simulink model "Luo_Converter_with_MOSFET"  (R2025a)
settings: Solver=VariableStepAuto  StartTime=0.0  StopTime=0.5  RelTol=1e-3
libraries: spsMeanLib x16, spsRMSLib x16, spsVoltageMeasurementLib x8, spsCurrentMeasurementLib x7, spsSeriesRLCBranchLib x5, spsDCVoltageSourceLib x1, spsDiodeLib x1, spsMosfetLib x1, sps_lib x1
settings Model: Creator=sanat  LastModifiedBy=sanat

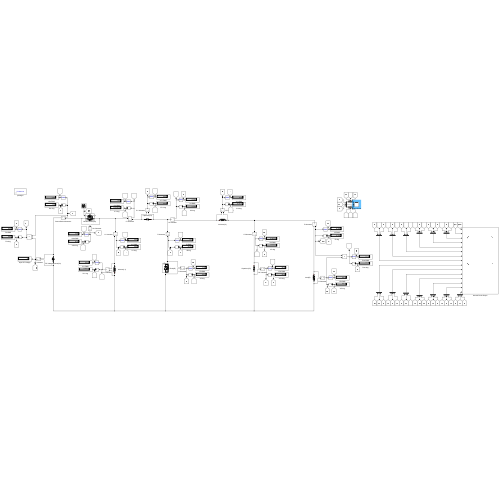
[thumbnail: Simulink's stored preview of the top-level diagram]
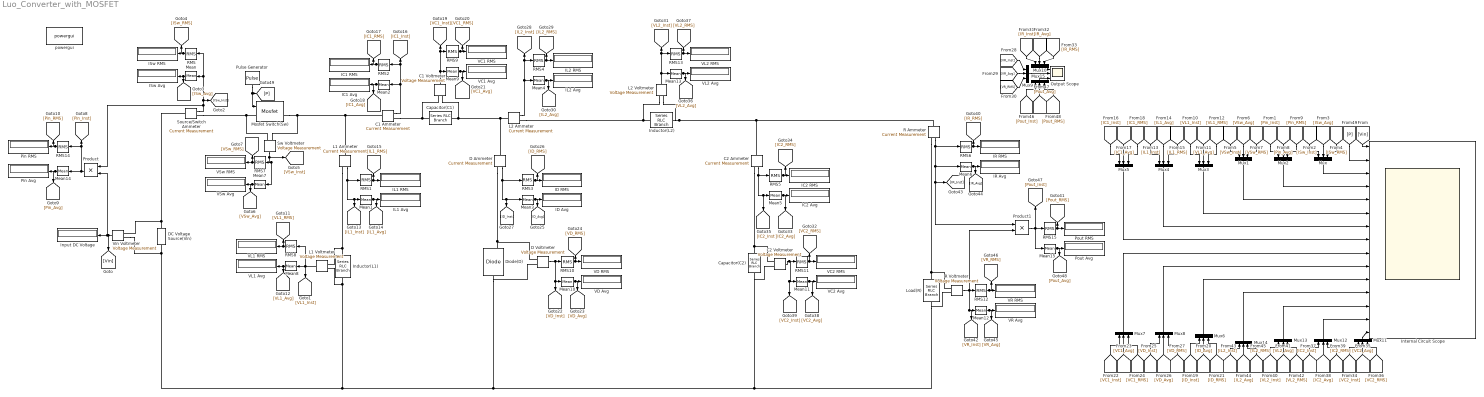
== system Luo_Converter_with_MOSFET ==
  C1 Ammeter : spsCurrentMeasurementLib/Current Measurement  PhasorSimulation=off  OutputType=Complex  PSBequivalent=0
  C1 Voltmeter : spsVoltageMeasurementLib/Voltage Measurement  PhasorSimulation=off  OutputType=Complex  PSBequivalent=0
  C2 Ammeter : spsCurrentMeasurementLib/Current Measurement  PhasorSimulation=off  OutputType=Complex  PSBequivalent=0
  C2 Voltmeter : spsVoltageMeasurementLib/Voltage Measurement  PhasorSimulation=off  OutputType=Complex  PSBequivalent=0
  Capacitor(C1) : spsSeriesRLCBranchLib/Series RLC Branch  LConnTagsString=__new0  RConnTagsString=__new0  BranchType=C  Resistance=1  Inductance=1e-3  SetiL0=off  InitialCurrent=0  Capacitance=21.40e-6  Setx0=off  InitialVoltage=0  Measurements=None
  Capacitor(C2) : spsSeriesRLCBranchLib/Series RLC Branch  LConnTagsString=__new0  RConnTagsString=__new0  BranchType=C  Resistance=1  Inductance=1e-3  SetiL0=off  InitialCurrent=0  Capacitance=30.4e-6  Setx0=off  InitialVoltage=0  Measurements=None
  D Ammeter : spsCurrentMeasurementLib/Current Measurement  PhasorSimulation=off  OutputType=Complex  PSBequivalent=0
  D Voltmeter : spsVoltageMeasurementLib/Voltage Measurement  PhasorSimulation=off  OutputType=Complex  PSBequivalent=0
  DC Voltage Source(Vin) : spsDCVoltageSourceLib/DC Voltage Source  Amplitude=40  Measurements=None
  Diode(D) : spsDiodeLib/Diode  Ron=0.001  Lon=0  Vf=0.8  IC=0  UseSnubber=0  Rs=500  Cs=250e-9  Measurements=on
  IC1 Avg : Display
  IC1 RMS : Display
  IC2 Avg : Display
  IC2 RMS : Display
  ID Avg : Display
  ID RMS : Display
  IL1 Avg : Display
  IL1 RMS : Display
  IL2 Avg : Display
  IL2 RMS : Display
  IR Avg : Display
  IR RMS : Display
  ISw Avg : Display
  ISw RMS : Display
  Inductor(L1) : spsSeriesRLCBranchLib/Series RLC Branch  LConnTagsString=__new0  RConnTagsString=__new0  BranchType=L  Resistance=1  Inductance=36.04e-3  SetiL0=off  InitialCurrent=0  Capacitance=1e-6  Setx0=off  InitialVoltage=0  Measurements=None
  Inductor(L2) : spsSeriesRLCBranchLib/Series RLC Branch  LConnTagsString=__new0  RConnTagsString=__new0  BranchType=L  Resistance=1  Inductance=36.04e-3  SetiL0=off  InitialCurrent=0  Capacitance=1e-6  Setx0=off  InitialVoltage=0  Measurements=None
  Input DC Voltage : Display
  Internal Circuit Scope : Scope  NumInputPorts=15
      settings: ActiveDisplayYMinimum=30  ActiveDisplayYMaximum=50  YLabel=Input Voltage
  L1 Ammeter : spsCurrentMeasurementLib/Current Measurement  PhasorSimulation=off  OutputType=Complex  PSBequivalent=0
  L1 Voltmeter : spsVoltageMeasurementLib/Voltage Measurement  PhasorSimulation=off  OutputType=Complex  PSBequivalent=0
  L2 Ammeter : spsCurrentMeasurementLib/Current Measurement  PhasorSimulation=off  OutputType=Complex  PSBequivalent=0
  L2 Voltmeter : spsVoltageMeasurementLib/Voltage Measurement  PhasorSimulation=off  OutputType=Complex  PSBequivalent=0
  Load(R) : spsSeriesRLCBranchLib/Series RLC Branch  LConnTagsString=__new0  RConnTagsString=__new0  BranchType=R  Resistance=135.2  Inductance=1e-3  SetiL0=off  InitialCurrent=0  Capacitance=1e-6  Setx0=off  InitialVoltage=0  Measurements=None
  Mean{,1..15} (16 alike) : spsMeanLib/Mean  Freq=60  Vinit=0  Ts=0
  Mosfet Switch(Sw) : spsMosfetLib/Mosfet  Ron=0.1  Lon=0  Rd=0.01  Vfd=0  IC=0  Rs=1e5  Cs=inf  Measurements=on
  Mux{,1..15} (16 alike) : Mux  Inputs=3
  Output Scope : Scope  NumInputPorts=3
      settings: ActiveDisplayYMinimum=0.728472  ActiveDisplayYMaximum=0.7284818  YLabel=Resistance(R) Current
  Pin Avg : Display
  Pin RMS : Display
  Pout Avg : Display
  Pout RMS : Display
  Product : Product
  Product1 : Product
  Pulse Generator : DiscretePulseGenerator  PulseType=Time based  Period=1/50000  PulseWidth=(5/7)*100
  R Ammeter : spsCurrentMeasurementLib/Current Measurement  PhasorSimulation=off  OutputType=Complex  PSBequivalent=0
  R Voltmeter : spsVoltageMeasurementLib/Voltage Measurement  PhasorSimulation=off  OutputType=Complex  PSBequivalent=0
  RMS{,1..15} (16 alike) : spsRMSLib/RMS  TrueRMS=on  Freq=60  RMSInit=120  Ts=0
  Source/Switch Ammeter : spsCurrentMeasurementLib/Current Measurement  PhasorSimulation=off  OutputType=Complex  PSBequivalent=0
  Sw Voltmeter : spsVoltageMeasurementLib/Voltage Measurement  PhasorSimulation=off  OutputType=Complex  PSBequivalent=0
  VC1 Avg : Display
  VC1 RMS : Display
  VC2 Avg : Display
  VC2 RMS : Display
  VD Avg : Display
  VD RMS : Display
  VL1 Avg : Display
  VL1 RMS : Display
  VL2 Avg : Display
  VL2 RMS : Display
  VR Avg : Display
  VR RMS : Display
  VSw Avg : Display
  VSw RMS : Display
  Vin Voltmeter : spsVoltageMeasurementLib/Voltage Measurement  PhasorSimulation=off  OutputType=Complex  PSBequivalent=0
  powergui : sps_lib/powergui  Priority=1  SimulationMode=Continuous  SampleTime=50e-6  frequency=60  Iterations=50  frequencyindice=0  Pbase=100e6  ErrMax=1e-4  UnitsV=kV  UnitsW=MW  buscounter=0  FunctionMessages=off  echomessages=off  EnableUseOfTLC=off  CurrentSourceSwitches=off  DisableSnubberDevices=off  DisableRonSwitches=off  DisableVfSwitches=off  DisplayEquations=off  AutomaticDiscreteSolvers=off  SolverType=Tustin/Backward Euler (TBE)  Interpol=off  ExternalGateDelay=off  methode=off  Ts=100  x0status=blocks  SPID=on  SwTol=0  HookPort=off  NonlinearTolerance=1e-4  nMaxIteration=100  ContinueOnMaxIteration=off  RestoreLinks=warning  ResistiveCurrentMeasurement=off  Frange=[0:2:500]  Ylog=off  Xlog=on  ShowGrid=off  save=off  variable=ZData  structure=0  ZoomFFT=off  StartTime=0.0  cycles=1  DisplayStyle=1  fundamental=60  FreqAxis=off  MaxFrequency=1000  frequencyindicesteady=1  RmsSteady=1  display=off
  wires:
  Pulse Generator/1 -> [P], Mosfet Switch(Sw)/1
  Vin Voltmeter/1 -> Product/2, Input DC Voltage/1, [Vin]
  L1 Ammeter/1 -> RMS1/1, [IL1_Inst], Mean1/1
  RMS1/1 -> [IL1_RMS], IL1 RMS/1
  Mean1/1 -> [IL1_Avg], IL1 Avg/1
  RMS/1 -> [ISw_RMS], ISw RMS/1
  Mean/1 -> [ISw_Avg], ISw Avg/1
  Source/Switch Ammeter/1 -> RMS/1, Mean/1, [ISw_Inst], Product/1
  RMS2/1 -> [IC1_RMS], IC1 RMS/1
  C1 Ammeter/1 -> [IC1_Inst], RMS2/1, Mean2/1
  Mean2/1 -> [IC1_Avg], IC1 Avg/1
  Mean3/1 -> [ID_Avg], ID Avg/1
  RMS3/1 -> [ID_RMS], ID RMS/1
  D Ammeter/1 -> [ID_Inst], Mean3/1, RMS3/1
  Mean4/1 -> [IL2_Avg], IL2 Avg/1
  RMS4/1 -> [IL2_RMS], IL2 RMS/1
  L2 Ammeter/1 -> [IL2_Inst], RMS4/1, Mean4/1
  RMS5/1 -> [IC2_RMS], IC2 RMS/1
  C2 Ammeter/1 -> RMS5/1, [IC2_Inst], Mean5/1
  Mean5/1 -> [IC2_Avg], IC2 Avg/1
  Mean6/1 -> [IR_Avg], IR Avg/1
  RMS6/1 -> [IR_RMS], IR RMS/1
  R Ammeter/1 -> Product1/1, [IR_Inst], Mean6/1, RMS6/1
  Mean7/1 -> [VSw_Avg], VSw Avg/1
  RMS7/1 -> [VSw_RMS], VSw RMS/1
  Mean8/1 -> [VL1_Avg], VL1 Avg/1
  L1 Voltmeter/1 -> [VL1_Inst], Mean8/1, RMS8/1
  RMS8/1 -> [VL1_RMS], VL1 RMS/1
  RMS9/1 -> [VC1_RMS], VC1 RMS/1
  Mean9/1 -> [VC1_Avg], VC1 Avg/1
  C1 Voltmeter/1 -> [VC1_Inst], RMS9/1, Mean9/1
  RMS10/1 -> [VD_RMS], VD RMS/1
  Mean10/1 -> [VD_Avg], VD Avg/1
  D Voltmeter/1 -> [VD_Inst], Mean10/1, RMS10/1
  Mean11/1 -> [VC2_Avg], VC2 Avg/1
  RMS11/1 -> [VC2_RMS], VC2 RMS/1
  C2 Voltmeter/1 -> [VC2_Inst], Mean11/1, RMS11/1
  Mean12/1 -> [VR_Avg], VR Avg/1
  RMS12/1 -> [VR_RMS], VR RMS/1
  R Voltmeter/1 -> Product1/2, [VR_Inst], Mean12/1, RMS12/1
  Mean13/1 -> [VL2_Avg], VL2 Avg/1
  RMS13/1 -> [VL2_RMS], VL2 RMS/1
  L2 Voltmeter/1 -> [VL2_Inst], RMS13/1, Mean13/1
  [ISw_Inst] -> Mux/1
  [ISw_Avg] -> Mux/2
  [ISw_RMS] -> Mux/3
  Sw Voltmeter/1 -> [VSw_Inst], RMS7/1, Mean7/1
  [VSw_Avg] -> Mux1/2
  [VSw_Inst] -> Mux1/1
  [VSw_RMS] -> Mux1/3
  RMS14/1 -> [Pin_RMS], Pin RMS/1
  Mean14/1 -> [Pin_Avg], Pin Avg/1
  Product/1 -> Mean14/1, RMS14/1, [Pin_Inst]
  [Pin_Avg] -> Mux2/2
  [Pin_Inst] -> Mux2/1
  [Pin_RMS] -> Mux2/3
  [VL1_Avg] -> Mux3/2
  [VL1_RMS] -> Mux3/3
  [VL1_Inst] -> Mux3/1
  [IL1_Avg] -> Mux4/2
  [IL1_RMS] -> Mux4/3
  [IL1_Inst] -> Mux4/1
  [IC1_RMS] -> Mux5/3
  [IC1_Avg] -> Mux5/2
  [IC1_Inst] -> Mux5/1
  [VC1_Avg] -> Mux7/2
  [VC1_Inst] -> Mux7/1
  [VC1_RMS] -> Mux7/3
  [VD_Avg] -> Mux8/2
  [VD_RMS] -> Mux8/3
  [VD_Inst] -> Mux8/1
  [ID_RMS] -> Mux6/3
  [ID_Inst] -> Mux6/1
  [ID_Avg] -> Mux6/2
  [VR_RMS] -> Mux9/3
  [VR_Inst] -> Mux9/1
  [VR_Avg] -> Mux9/2
  [IR_RMS] -> Mux10/3
  [IR_Avg] -> Mux10/2
  [IR_Inst] -> Mux10/1
  [VC2_RMS] -> Mux11/3
  [VC2_Avg] -> Mux11/2
  [VC2_Inst] -> Mux11/1
  [IC2_RMS] -> Mux12/3
  [IC2_Avg] -> Mux12/2
  [IC2_Inst] -> Mux12/1
  [VL2_RMS] -> Mux13/3
  [VL2_Avg] -> Mux13/2
  [VL2_Inst] -> Mux13/1
  [IL2_RMS] -> Mux14/3
  [IL2_Avg] -> Mux14/2
  [IL2_Inst] -> Mux14/1
  Mean15/1 -> [Pout_Avg], Pout Avg/1
  RMS15/1 -> [Pout_RMS], Pout RMS/1
  Product1/1 -> Mean15/1, [Pout_Inst], RMS15/1
  [Pout_RMS] -> Mux15/3
  [Pout_Inst] -> Mux15/1
  [Pout_Avg] -> Mux15/2
  Mux15/1 -> Output Scope/3
  Mux9/1 -> Output Scope/2
  Mux10/1 -> Output Scope/1
  [Vin] -> Internal Circuit Scope/1
  [P] -> Internal Circuit Scope/2
  Mux/1 -> Internal Circuit Scope/3
  Mux2/1 -> Internal Circuit Scope/4
  Mux1/1 -> Internal Circuit Scope/5
  Mux11/1 -> Internal Circuit Scope/15
  Mux12/1 -> Internal Circuit Scope/14
  Mux13/1 -> Internal Circuit Scope/13
  Mux14/1 -> Internal Circuit Scope/12
  Mux3/1 -> Internal Circuit Scope/6
  Mux4/1 -> Internal Circuit Scope/7
  Mux5/1 -> Internal Circuit Scope/8
  Mux8/1 -> Internal Circuit Scope/10
  Mux6/1 -> Internal Circuit Scope/11
  Mux7/1 -> Internal Circuit Scope/9
  connections:
  DC Voltage Source(Vin)/RConn1 -- Source/Switch Ammeter/LConn1 -- Vin Voltmeter/LConn1
  Mosfet Switch(Sw)/RConn1 -- Sw Voltmeter/LConn2 -- C1 Ammeter/LConn1 -- L1 Ammeter/LConn1
  Inductor(L1)/LConn1 -- L1 Voltmeter/LConn2 -- D Voltmeter/LConn1 -- Diode(D)/LConn1 -- R Voltmeter/LConn2 -- Load(R)/RConn1 -- C2 Voltmeter/LConn2 -- Capacitor(C2)/RConn1 -- Vin Voltmeter/LConn2 -- DC Voltage Source(Vin)/LConn1
  Capacitor(C1)/LConn1 -- C1 Voltmeter/LConn1 -- L2 Ammeter/LConn1 -- D Ammeter/LConn1
  Inductor(L2)/RConn1 -- R Ammeter/LConn1 -- C2 Ammeter/LConn1 -- L2 Voltmeter/LConn2
  C1 Ammeter/RConn1 -- C1 Voltmeter/LConn2 -- Capacitor(C1)/RConn1
  Source/Switch Ammeter/RConn1 -- Sw Voltmeter/LConn1 -- Mosfet Switch(Sw)/LConn1
  L1 Ammeter/RConn1 -- L1 Voltmeter/LConn1 -- Inductor(L1)/RConn1
  D Ammeter/RConn1 -- D Voltmeter/LConn2 -- Diode(D)/RConn1
  L2 Ammeter/RConn1 -- L2 Voltmeter/LConn1 -- Inductor(L2)/LConn1
  C2 Ammeter/RConn1 -- C2 Voltmeter/LConn1 -- Capacitor(C2)/LConn1
  R Ammeter/RConn1 -- R Voltmeter/LConn1 -- Load(R)/LConn1
